simulink model "physicssim"  (R2019b)
settings: Solver=VariableStepAuto  StartTime=0.0  StopTime=3  RelTol=1e-3
values from neighbouring files (symbols this model uses):
  x0 = [0, 0, 0.05, 2, 0, 0.01, 0.02, 0, 0, 0, 0, 0]    [createmodels.m]    (also in pidcontrolstartupscript.m = [0, 0, 0.05, 8, 0, 0.01, 0.02, 0, 0, 0, 0, 0])
undefined symbols (not defined in the file or in its folder): scalemodelstatefunction
libraries: aerolibanim x1
settings Model: PacingRate=0.110000  Creator=Vlad  LastModifiedBy=Vlad

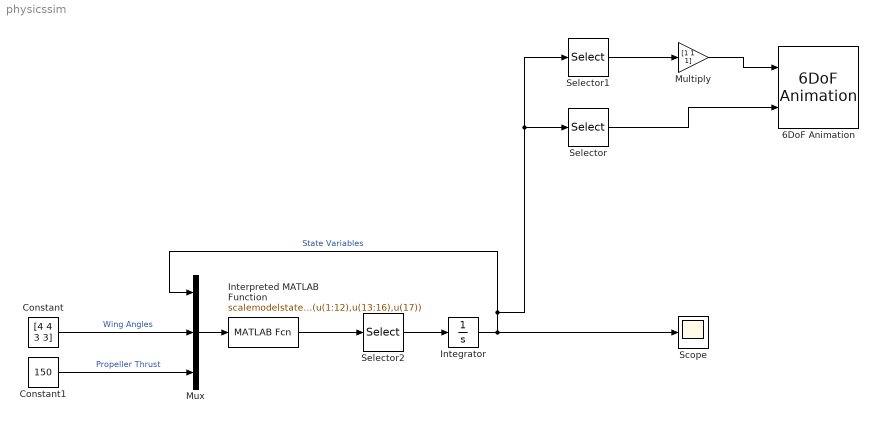
== system physicssim ==
  6DoF Animation : aerolibanim/6DoF Animation  u1=[0 30 -2 2 -1 0]  u2=0.1  u3=5  u4=[4000 0 -5000]  u5=Fly alongside  u6=[20 20 -20]  u7=20  u8=on
      settings: SourceProductName=Aerospace Blockset
  Constant : Constant  Value=[4 4 3 3]
  Constant1 : Constant  Value=150
  Integrator : Integrator  InitialCondition=x0
  Interpreted MATLAB Function : MATLABFcn  MATLABFcn=scalemodelstatefunction(u(1:12),u(13:16),u(17))  OutputDimensions=12
  Multiply : Gain  Gain=[1 1 1]
  Mux : Mux  Inputs=3
  Scope : Scope
  Selector : Selector  InputPortWidth=12  IndexOptions=Index vector (dialog)  Indices=[8 7 9]  OutputSizes=1
  Selector1 : Selector  InputPortWidth=12  IndexOptions=Index vector (dialog)  Indices=[1 2 3]  OutputSizes=1
  Selector2 : Selector  InputPortWidth=12  IndexOptions=Index vector (dialog)  Indices=[1 2 3 4 5 6 7 8 9 10 11 12]  OutputSizes=1
  wires:
  Selector1/1 -> Multiply/1
  Selector/1 -> 6DoF Animation/2
  Integrator/1 -> Scope/1, Selector/1, Selector1/1, Mux/1  "State Variables"
  Multiply/1 -> 6DoF Animation/1
  Constant1/1 -> Mux/3  "Propeller Thrust"
  Constant/1 -> Mux/2  "Wing Angles"
  Mux/1 -> Interpreted MATLAB Function/1
  Interpreted MATLAB Function/1 -> Selector2/1
  Selector2/1 -> Integrator/1
